simulink model "wastegate_img"  (R2012b)
settings: Solver=ode45  StartTime=0.0  StopTime=10.0  RelTol=1e-3
values from neighbouring files (symbols this model uses):
  A_max_wg = 0.035^2/4*pi    (= 0.000962112750162)    [Init_Project2.m]
  Cd_wg = 0.9    [Init_Project2.m]
  gamma_exh = 1.4    [Init_Project1.m]
  tau_wg = 1    [Init_Project2.m]
undefined symbols (not defined in the file or in its folder): Newton, Raphson
settings Model: Creator=rasme879  LastModifiedBy=rasme879

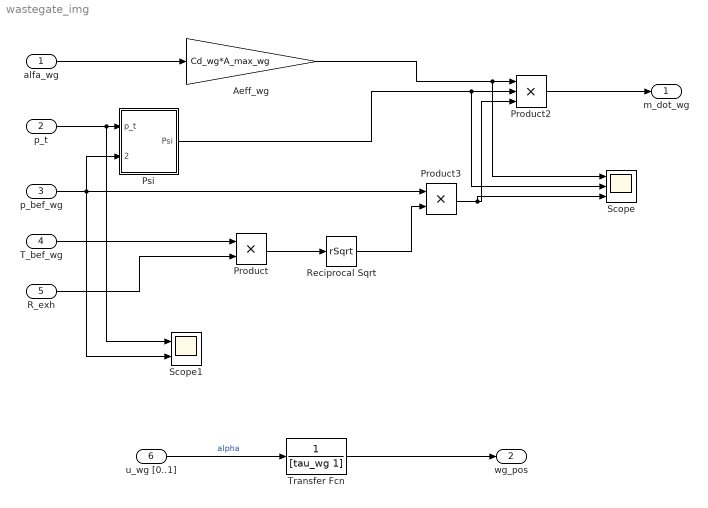
== system wastegate_img ==
  alfa_wg : Inport
  p_t : Inport  Port=2
  p_bef_wg : Inport  Port=3
  T_bef_wg : Inport  Port=4
  R_exh : Inport  Port=5
  u_wg [0..1] : Inport  Port=6
  Aeff_wg : Gain  Gain=Cd_wg*A_max_wg
  Product : Product
  Product2 : Product  Inputs=3  RndMeth=Zero
  Product3 : Product  RndMeth=Zero
  Psi : Subsystem
  Reciprocal Sqrt : Sqrt  Operator=rSqrt  SaturateOnIntegerOverflow=on
  Scope : Scope  NumInputPorts=3
      settings: YMin=-5~-5~-5  YMax=5~5~5
  Scope1 : Scope  NumInputPorts=2
      settings: YMin=-5~-5  YMax=5~5
  Transfer Fcn : TransferFcn  Denominator=[tau_wg 1]
  m_dot_wg : Outport
  wg_pos : Outport  Port=2
  wires:
  p_bef_wg/1 -> Scope1/2, Product3/1, Psi/2(p_bef_wg)
  Psi/1(Psi) -> Scope/2, Product2/2
  Aeff_wg/1 -> Scope/1, Product2/1
  Product3/1 -> Scope/3, Product2/3
  Reciprocal Sqrt/1 -> Product3/2
  Product/1 -> Reciprocal Sqrt/1
  alfa_wg/1 -> Aeff_wg/1
  Product2/1 -> m_dot_wg/1
  p_t/1 -> Scope1/1, Psi/1(p_t)
  T_bef_wg/1 -> Product/1
  R_exh/1 -> Product/2
  u_wg [0..1]/1 -> Transfer Fcn/1  "alpha"
  Transfer Fcn/1 -> wg_pos/1

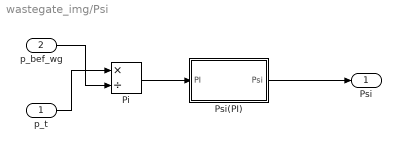
== system wastegate_img/Psi ==
  p_t : Inport
  p_bef_wg : Inport  Port=2
  Pi : Product  Inputs=*/
  Psi(PI) : Subsystem
  Psi : Outport
  wires:
  Pi/1 -> Psi(PI)/1(PI)
  Psi(PI)/1(Psi) -> Psi/1
  p_t/1 -> Pi/1
  p_bef_wg/1 -> Pi/2

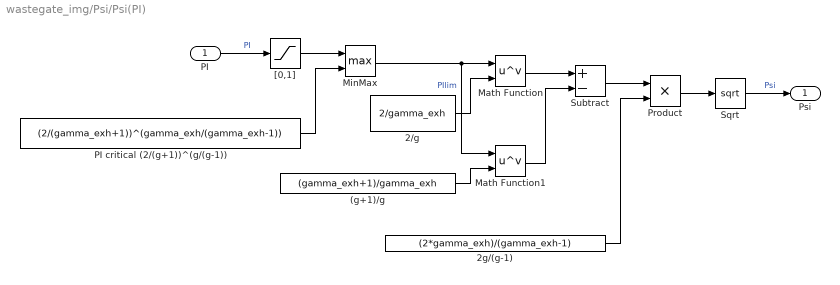
== system wastegate_img/Psi/Psi(PI) ==
  PI : Inport
  (g+1)/g : Constant  Value=(gamma_exh+1)/gamma_exh
  2/g : Constant  Value=2/gamma_exh
  2g/(g-1) : Constant  Value=(2*gamma_exh)/(gamma_exh-1)
  Math Function : Math  Operator=pow  SaturateOnIntegerOverflow=on
  Math Function1 : Math  Operator=pow  SaturateOnIntegerOverflow=on
  MinMax : MinMax  Function=max  Inputs=2
  PI critical (2/(g+1))^(g/(g-1)) : Constant  Value=(2/(gamma_exh+1))^(gamma_exh/(gamma_exh-1))
  Product : Product  RndMeth=Zero
  Sqrt : Sqrt  AlgorithmType=Newton-Raphson  SaturateOnIntegerOverflow=on
  Subtract : Sum  Inputs=+-
  "[0,1]" : Saturate  UpperLimit=1  LowerLimit=0
  Psi : Outport
  wires:
  PI/1 -> "[0,1]"/1  "PI"
  PI critical (2/(g+1))^(g/(g-1))/1 -> MinMax/2
  MinMax/1 -> Math Function/1, Math Function1/1  "PIlim"
  2/g/1 -> Math Function/2
  (g+1)/g/1 -> Math Function1/2
  "[0,1]"/1 -> MinMax/1
  Math Function/1 -> Subtract/1
  Math Function1/1 -> Subtract/2
  Subtract/1 -> Product/1
  2g/(g-1)/1 -> Product/2
  Product/1 -> Sqrt/1
  Sqrt/1 -> Psi/1  "Psi"
